simulink model "full_model_simulated"  (R2020a)
settings: Solver=VariableStepAuto  StartTime=0.0  StopTime=ref(end,1)  RelTol=1e-3
values from neighbouring files (symbols this model uses):
  alpha1hat = 0.0114    [Linearize_whitebox.m]    (also in Linearize_whitebox_final.m; lqr_whitebox.mat; matrices.mat)
  alpha2hat = 0.0079    [Linearize_whitebox.m]    (also in Linearize_whitebox_final.m; lqr_whitebox.mat; matrices.mat)
  areahat = 0.0009    [Linearize_whitebox.m]    (also in Linearize_whitebox_final.m; lqr_whitebox.mat; matrices.mat)
  areashat = 0.0004    [Linearize_whitebox.m]    (also in Linearize_whitebox_final.m; lqr_whitebox.mat; matrices.mat)
  boltz = 5.67e-8    (= 5.67e-08)    [Linearize_whitebox.m]    (also in Linearize_whitebox_final.m; lqr_whitebox.mat; matrices.mat; nonlinid.m)
  C = Ad.C    [Observer_mat.m]    (also in discretemodel.mat = [0  0  1  0; 0  0  0  1]; lqr_whitebox.m = sys.C; lqr_whitebox.mat = [0  0  1  0; 0  0  0  1]; matrices.mat = [0  0  1  0; 0  0  0  1])
  cphat = 501.9208    [Linearize_whitebox.m]    (also in Linearize_whitebox_final.m; lqr_whitebox.mat; matrices.mat)
  emishat = 0.9000    (= 0.9)    [Linearize_whitebox.m]    (also in Linearize_whitebox_final.m; lqr_whitebox.mat; matrices.mat)
  gamma = Ad.B    [Observer_mat.m]    (also in discretemodel.mat = [0.004353030085  4.48398112985e-06; 6.47055504813e-06  0.003; observer_matlab.m; observermatlab.m)
  h = tout(2)-tout(1)    [Linearize_whitebox.m]    (also in Linearize_whitebox_final.m; Observer_mat.m; lqr_whitebox.mat = 1.00037043897; matrices.mat = 1.00080032013)
  K = [0.871464143609  0.0262786205748; 0.0262786205748  0.871464143609; 0.341518856741  0.00295216925623; 0.00295216925623  0.341518856741]    [K_matrix.mat]    (also in K_matrix_final.mat = [0.107540648809  0.00297468629139; 0.00297468629139  0.10754; Observer_mat.m = place(phi.',C.',P).'; lqr_whitebox.m = lqr(A,B,Q,R); lqr_whitebox.mat = [9.8403850338  0.823629600444  7.09136571585  0.104667034235)
  L = lqr(A,B,Q,R)    [LQR.m]    (also in LQR_final.m; L_Lr_LQR.mat = [210.936834033  1.0429491506  82.9532479278  0.141237062686;; L_Lr_LQR_final.mat = [15.3959700225  0.0810970521206  45.9635678787  0.9358925165; L_Lr_Pole_Placement.mat = [382.498734136  0.681043508792  3740.11964319  0; 0.98277164)
  Lr = inv(Ldc)    [LQR.m]    (also in LQR_final.m; L_Lr_LQR.mat = [295.811652311  0.50314270449; -0.353029029898  433.02182351; L_Lr_LQR_final.mat = [63.2811082521  0.33594605992; -0.399513584683  63.309082518; L_Lr_Pole_Placement.mat = [4124.53994767  0; 0  5951.86777259])
  masshat = 0.0052    [Linearize_whitebox.m]    (also in Linearize_whitebox_final.m; lqr_whitebox.mat; matrices.mat)
  phi = Ad.A    [Observer_mat.m]    (also in discretemodel.mat = [0.991639753181 0.00295216925623 0.0399517774449 5.979211225; observer_matlab.m; observermatlab.m)
  tauhat = 24.4408    [Linearize_whitebox.m]    (also in Linearize_whitebox_final.m; lqr_whitebox.mat; matrices.mat)
  u0 = [15; 15]    [observer_matlab.m]
  uhat = 10.2021    [Linearize_whitebox.m]    (also in Linearize_whitebox_final.m; lqr_whitebox.mat; matrices.mat)
  ushat = 13.8985    [Linearize_whitebox.m]    (also in Linearize_whitebox_final.m; lqr_whitebox.mat; matrices.mat)
  y0 = [300; 300]    [observer_matlab.m]
undefined symbols (not defined in the file or in its folder): init_temp
libraries: simulink x1
settings Model: Creator=SIDTUDelft1  LastModifiedBy=SIDTUDelft1

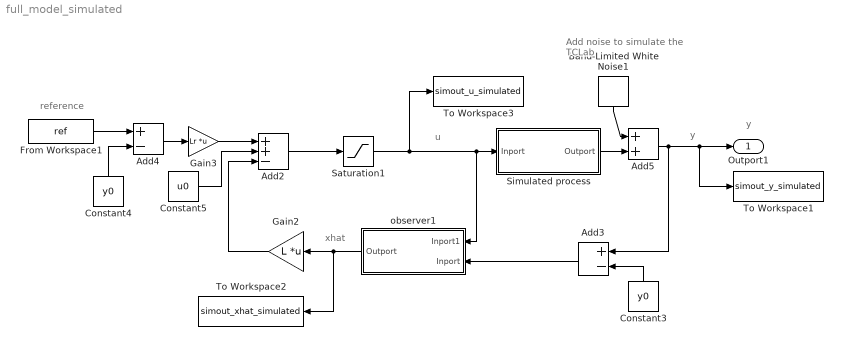
== system full_model_simulated ==
  note: Add noise to simulate
      | the TCLab
  note: y
  note: u
  note: reference
  note: xhat
  note: y
  Add2 : Sum  Inputs=++-  OutMin=[0]  OutMax=[100]
  Add3 : Sum  Inputs=+-
  Add4 : Sum  Inputs=+-
  Add5 : Sum
  Band-Limited White Noise1 : simulink/Sources/Band-Limited White Noise  Cov=[0.5]  Ts=h  seed=[23341]
  Constant3 : Constant  Value=y0
  Constant4 : Constant  Value=y0
  Constant5 : Constant  Value=u0  SampleTime=h
  From Workspace1 : FromWorkspace  VariableName=ref  SampleTime=h
  Gain2 : Gain  Gain=L  Multiplication=Matrix(K*u)
  Gain3 : Gain  Gain=Lr  Multiplication=Matrix(K*u)
  Saturation1 : Saturate  UpperLimit=100  LowerLimit=0
  Simulated process : Subsystem
  To Workspace1 : ToWorkspace  VariableName=simout_y_simulated  SaveFormat=Timeseries  SampleTime=-1
  To Workspace2 : ToWorkspace  VariableName=simout_xhat_simulated  SaveFormat=Timeseries  SampleTime=-1
  To Workspace3 : ToWorkspace  VariableName=simout_u_simulated  SaveFormat=Timeseries  SampleTime=-1
  observer1 : Subsystem
  Outport1 : Outport
  wires:
  observer1/1(Outport) -> Gain2/1, To Workspace2/1
  Constant4/1 -> Add4/2
  Add4/1 -> Gain3/1
  Saturation1/1 -> Simulated process/1(Inport), observer1/1(Inport1), To Workspace3/1
  Add3/1 -> observer1/2(Inport)
  Constant5/1 -> Add2/2
  Gain2/1 -> Add2/3
  Constant3/1 -> Add3/2
  Gain3/1 -> Add2/1
  From Workspace1/1 -> Add4/1
  Add2/1 -> Saturation1/1
  Band-Limited White Noise1/1 -> Add5/1
  Simulated process/1(Outport) -> Add5/2
  Add5/1 -> To Workspace1/1, Outport1/1, Add3/1

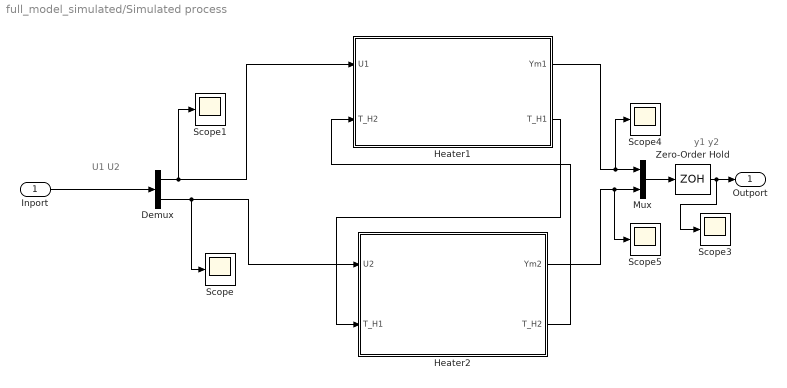
== system full_model_simulated/Simulated process ==
  note: y1 y2
  note: U1 U2
  Inport : Inport
  Demux : Demux  Outputs=2
  Heater1 : Subsystem
  Heater2 : Subsystem
  Mux : Mux  Inputs=2
  Scope{,1,3..5} (5 alike) : Scope
  Zero-Order Hold : ZeroOrderHold  SampleTime=h
  Outport : Outport
  wires:
  Heater2/1(Ym2) -> Mux/2, Scope5/1
  Heater1/2(T_H1) -> Heater2/2(T_H1)
  Heater2/2(T_H2) -> Heater1/2(T_H2)
  Heater1/1(Ym1) -> Scope4/1, Mux/1
  Demux/1 -> Heater1/1(U1), Scope1/1
  Demux/2 -> Scope/1, Heater2/1(U2)
  Mux/1 -> Zero-Order Hold/1
  Inport/1 -> Demux/1
  Zero-Order Hold/1 -> Scope3/1, Outport/1

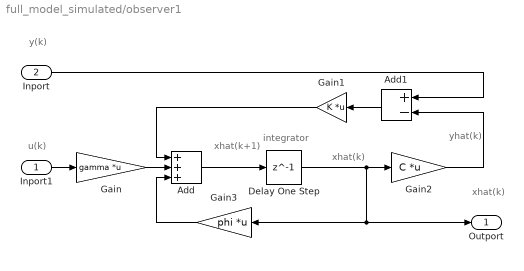
== system full_model_simulated/observer1 ==
  note: yhat(k)
  note: xhat(k+1)
  note: y(k)
  note: xhat(k)
  note: u(k)
  note: xhat(k)
  note: integrator
  Inport1 : Inport
  Inport : Inport  Port=2
  Add : Sum  Inputs=+++
  Add1 : Sum  Inputs=+-
  Delay One Step : Delay  DelayLength=1  SampleTime=h
  Gain : Gain  Gain=gamma  Multiplication=Matrix(K*u)
  Gain1 : Gain  Gain=K  Multiplication=Matrix(K*u)
  Gain2 : Gain  Gain=C  Multiplication=Matrix(K*u)
  Gain3 : Gain  Gain=phi  Multiplication=Matrix(K*u)
  Outport : Outport
  wires:
  Add/1 -> Delay One Step/1
  Add1/1 -> Gain1/1
  Gain1/1 -> Add/1
  Gain/1 -> Add/2
  Gain2/1 -> Add1/2
  Gain3/1 -> Add/3
  Inport/1 -> Add1/1
  Inport1/1 -> Gain/1
  Delay One Step/1 -> Gain3/1, Outport/1, Gain2/1

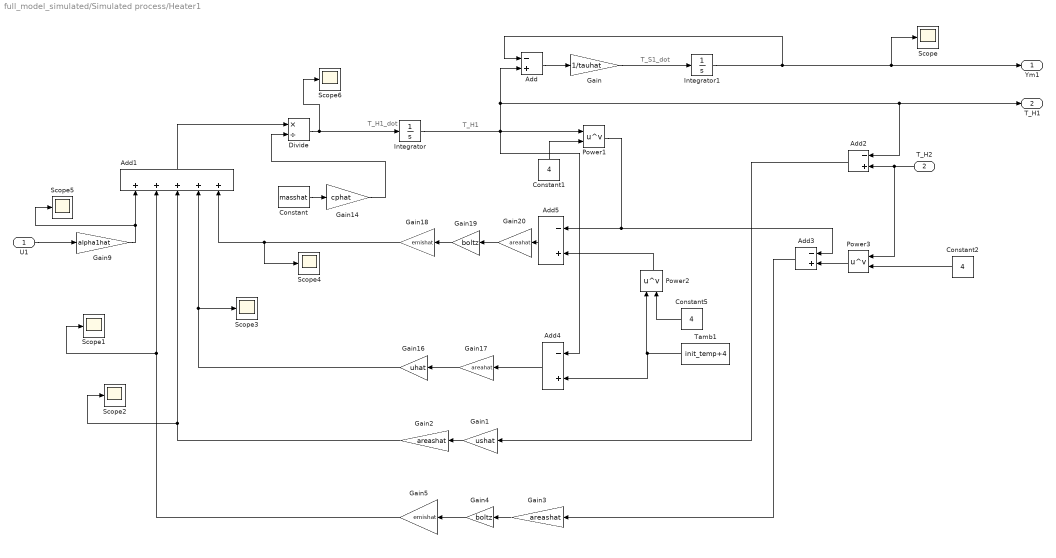
== system full_model_simulated/Simulated process/Heater1 ==
  note: T_S1_dot
  note: T_H1
  note: T_H1_dot
  U1 : Inport
  T_H2 : Inport  Port=2
  Add{,2..5} (5 alike) : Sum  Inputs=-+
  Add1 : Sum  Inputs=+++++
  Constant : Constant  Value=masshat
  Constant1 : Constant  Value=4
  Constant2 : Constant  Value=4
  Constant5 : Constant  Value=4
  Divide : Product  Inputs=*/
  Gain : Gain  Gain=1/tauhat
  Gain1 : Gain  Gain=ushat
  Gain14 : Gain  Gain=cphat
  Gain16 : Gain  Gain=uhat
  Gain17 : Gain  Gain=areahat
  Gain18 : Gain  Gain=emishat
  Gain19 : Gain  Gain=boltz
  Gain2 : Gain  Gain=areashat
  Gain20 : Gain  Gain=areahat
  Gain3 : Gain  Gain=areashat
  Gain4 : Gain  Gain=boltz
  Gain5 : Gain  Gain=emishat
  Gain9 : Gain  Gain=alpha1hat
  Integrator : Integrator  InitialCondition=init_temp
  Integrator1 : Integrator  InitialCondition=init_temp
  Power1 : Math  Operator=pow  SaturateOnIntegerOverflow=on
  Power2 : Math  Operator=pow  SaturateOnIntegerOverflow=on
  Power3 : Math  Operator=pow  SaturateOnIntegerOverflow=on
  Scope{,1..6} (7 alike) : Scope
  Tamb1 : Constant  Value=init_temp+4  SampleTime=h
  Ym1 : Outport
  T_H1 : Outport  Port=2
  wires:
  Add/1 -> Gain/1
  Gain17/1 -> Gain16/1
  Constant5/1 -> Power2/2
  Constant1/1 -> Power1/2
  Add5/1 -> Gain20/1
  Add1/1 -> Divide/1
  Add4/1 -> Gain17/1
  Gain20/1 -> Gain19/1
  Tamb1/1 -> Add4/2, Power2/1
  Divide/1 -> Integrator/1, Scope6/1
  Power2/1 -> Add5/2
  Power1/1 -> Add3/1, Add5/1
  Gain19/1 -> Gain18/1
  Gain18/1 -> Scope4/1, Add1/5
  Gain9/1 -> Add1/1, Scope5/1
  Gain16/1 -> Scope3/1, Add1/4
  Gain1/1 -> Gain2/1
  T_H2/1 -> Power3/1, Add2/2
  Add2/1 -> Gain1/1
  Gain2/1 -> Add1/3, Scope2/1
  Constant2/1 -> Power3/2
  Power3/1 -> Add3/2
  Gain4/1 -> Gain5/1
  Gain3/1 -> Gain4/1
  Add3/1 -> Gain3/1
  Gain5/1 -> Scope1/1, Add1/2
  Constant/1 -> Gain14/1
  Gain14/1 -> Divide/2
  Gain/1 -> Integrator1/1
  Integrator1/1 -> Add/1, Scope/1, Ym1/1
  U1/1 -> Gain9/1
  Integrator/1 -> Add4/1, Add2/1, T_H1/1, Add/2, Power1/1

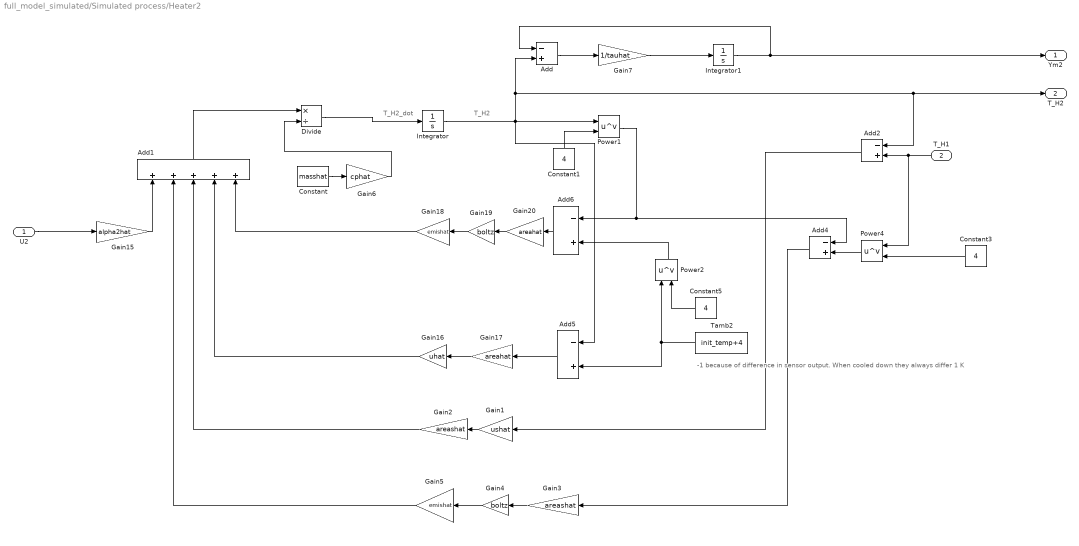
== system full_model_simulated/Simulated process/Heater2 ==
  note: -1 because of difference in sensor output. When cooled down they always differ 1 K
  note: T_H2
  note: T_H2_dot
  U2 : Inport
  T_H1 : Inport  Port=2
  Add{,2,4..6} (5 alike) : Sum  Inputs=-+
  Add1 : Sum  Inputs=+++++
  Constant : Constant  Value=masshat
  Constant1 : Constant  Value=4
  Constant3 : Constant  Value=4
  Constant5 : Constant  Value=4
  Divide : Product  Inputs=*/
  Gain1 : Gain  Gain=ushat
  Gain15 : Gain  Gain=alpha2hat
  Gain16 : Gain  Gain=uhat
  Gain17 : Gain  Gain=areahat
  Gain18 : Gain  Gain=emishat
  Gain19 : Gain  Gain=boltz
  Gain2 : Gain  Gain=areashat
  Gain20 : Gain  Gain=areahat
  Gain3 : Gain  Gain=areashat
  Gain4 : Gain  Gain=boltz
  Gain5 : Gain  Gain=emishat
  Gain6 : Gain  Gain=cphat
  Gain7 : Gain  Gain=1/tauhat
  Integrator : Integrator  InitialCondition=init_temp
  Integrator1 : Integrator  InitialCondition=init_temp
  Power1 : Math  Operator=pow  SaturateOnIntegerOverflow=on
  Power2 : Math  Operator=pow  SaturateOnIntegerOverflow=on
  Power4 : Math  Operator=pow  SaturateOnIntegerOverflow=on
  Tamb2 : Constant  Value=init_temp+4  SampleTime=h
  Ym2 : Outport
  T_H2 : Outport  Port=2
  wires:
  Gain17/1 -> Gain16/1
  Power4/1 -> Add4/2
  Gain20/1 -> Gain19/1
  Tamb2/1 -> Add5/2, Power2/1
  Constant3/1 -> Power4/2
  Integrator/1 -> Add5/1, T_H2/1, Add2/1, Add/2, Power1/1
  Add6/1 -> Gain20/1
  Gain1/1 -> Gain2/1
  Add4/1 -> Gain3/1
  Gain18/1 -> Add1/5
  Power2/1 -> Add6/2
  Add/1 -> Gain7/1
  Gain4/1 -> Gain5/1
  Constant1/1 -> Power1/2
  Add2/1 -> Gain1/1
  Constant5/1 -> Power2/2
  Add5/1 -> Gain17/1
  Gain2/1 -> Add1/3
  Gain5/1 -> Add1/2
  T_H1/1 -> Power4/1, Add2/2
  Divide/1 -> Integrator/1
  Gain19/1 -> Gain18/1
  Gain16/1 -> Add1/4
  Gain3/1 -> Gain4/1
  Gain15/1 -> Add1/1
  U2/1 -> Gain15/1
  Gain6/1 -> Divide/2
  Constant/1 -> Gain6/1
  Add1/1 -> Divide/1
  Gain7/1 -> Integrator1/1
  Integrator1/1 -> Add/1, Ym2/1
  Power1/1 -> Add4/1, Add6/1
